simulink model "PLCCylinderCascade"  (R2020a)
settings: Solver=VariableStepAuto  StartTime=0.0  StopTime=inf  RelTol=1e-3
libraries: library_plc2simulink x27
settings Model: EnablePacing=on  Creator=Moritz  LastModifiedBy=Moritz

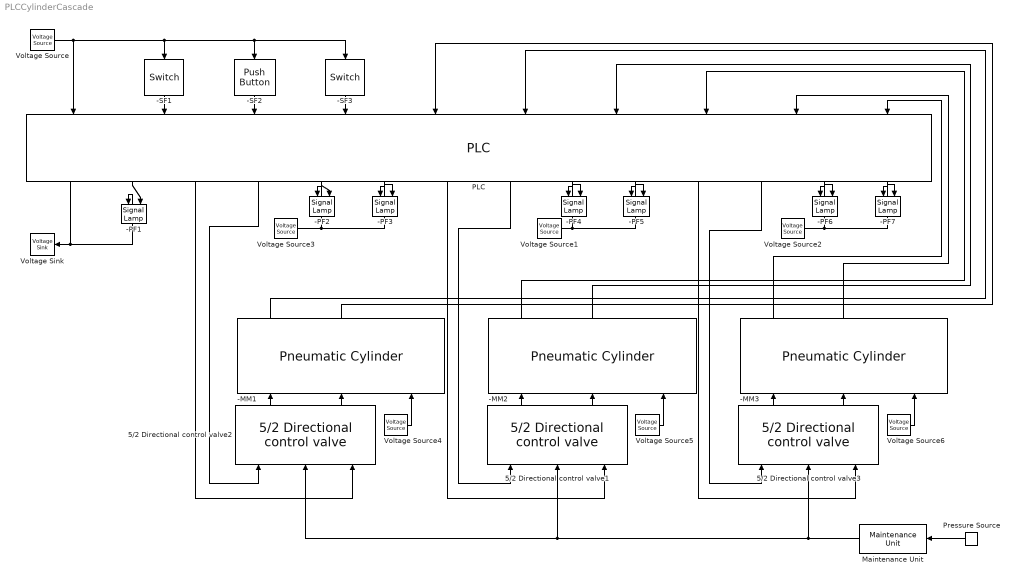
== system PLCCylinderCascade ==
  -MM1 : library_plc2simulink/Pneumatic Cylinder  minPos=0  maxPos=100  pistonSpeed=200  currentPos=-2.3002e-28  updateIcon=0.1
      settings: SourceProductName=PLC2Simulink
  -MM2 : library_plc2simulink/Pneumatic Cylinder  minPos=0  maxPos=100  pistonSpeed=200  currentPos=-2.3002e-28  updateIcon=0.1
      settings: SourceProductName=PLC2Simulink
  -MM3 : library_plc2simulink/Pneumatic Cylinder  minPos=0  maxPos=100  pistonSpeed=200  currentPos=-2.3002e-28  updateIcon=0.1
      settings: SourceProductName=PLC2Simulink
  -PF1 : library_plc2simulink/Signal Lamp  Value=off  updateTime=0.1  colorOn=[0.2,1,0.2]  colorOff=[1,1,1]
      settings: SourceProductName=PLC2Simulink
  -PF2 : library_plc2simulink/Signal Lamp  Value=on  updateTime=0.1  colorOn=[0.2,1,0.2]  colorOff=[1,1,1]
      settings: SourceProductName=PLC2Simulink
  -PF3 : library_plc2simulink/Signal Lamp  Value=off  updateTime=0.1  colorOn=[1,1,0.2]  colorOff=[1,1,1]
      settings: SourceProductName=PLC2Simulink
  -PF4 : library_plc2simulink/Signal Lamp  Value=on  updateTime=0.1  colorOn=[0.2,1,0.2]  colorOff=[1,1,1]
      settings: SourceProductName=PLC2Simulink
  -PF5 : library_plc2simulink/Signal Lamp  Value=off  updateTime=0.1  colorOn=[1,1,0.2]  colorOff=[1,1,1]
      settings: SourceProductName=PLC2Simulink
  -PF6 : library_plc2simulink/Signal Lamp  Value=on  updateTime=0.1  colorOn=[0.2,1,0.2]  colorOff=[1,1,1]
      settings: SourceProductName=PLC2Simulink
  -PF7 : library_plc2simulink/Signal Lamp  Value=off  updateTime=0.1  colorOn=[1,1,0.2]  colorOff=[1,1,1]
      settings: SourceProductName=PLC2Simulink
  -SF1 : library_plc2simulink/Switch  Gain=0  Multiplication=Element-wise(K.*u)  ParamMin=[]  ParamMax=[]  OutMin=[]  OutMax=[]  SampleTime=-1
      settings: SourceProductName=PLC2Simulink
  -SF2 : library_plc2simulink/Push Button  deactTime=0.3  StateOn=0
      settings: SourceProductName=PLC2Simulink
  -SF3 : library_plc2simulink/Switch  Gain=0  Multiplication=Element-wise(K.*u)  ParamMin=[]  ParamMax=[]  OutMin=[]  OutMax=[]  SampleTime=-1
      settings: SourceProductName=PLC2Simulink
  5/2 Directional control valve1 : library_plc2simulink/5//2 Directional control valve  updateIcon=0.1  state=0
      settings: SourceProductName=PLC2Simulink
  5/2 Directional control valve2 : library_plc2simulink/5//2 Directional control valve  updateIcon=0.1  state=0
      settings: SourceProductName=PLC2Simulink
  5/2 Directional control valve3 : library_plc2simulink/5//2 Directional control valve  updateIcon=0.1  state=0
      settings: SourceProductName=PLC2Simulink
  Maintenance Unit : library_plc2simulink/Maintenance Unit  pressure=0.300
      settings: SourceProductName=PLC2Simulink
  PLC : library_plc2simulink/PLC  instanceName=PLC1  numInputs=9  numOutputs=13  timeStep=0.05  externalSupplyVoltage=on
      settings: SourceProductName=PLC2Simulink
  Pressure Source : library_plc2simulink/Pressure Source  pressure=5
      settings: SourceProductName=PLC2Simulink
  Voltage Sink : library_plc2simulink/Voltage Sink
      settings: SourceProductName=PLC2Simulink
  Voltage Source{,4..6} (4 alike) : library_plc2simulink/Voltage Source  voltage=24
      settings: SourceProductName=PLC2Simulink
  Voltage Source1 : library_plc2simulink/Voltage Source  voltage=0
      settings: SourceProductName=PLC2Simulink
  Voltage Source2 : library_plc2simulink/Voltage Source  voltage=0
      settings: SourceProductName=PLC2Simulink
  Voltage Source3 : library_plc2simulink/Voltage Source  voltage=0
      settings: SourceProductName=PLC2Simulink
  wires:
  Pressure Source/1 -> Maintenance Unit/1
  -SF3/1 -> PLC/4
  Voltage Source/1 -> -SF3/1, -SF2/1, -SF1/1, PLC/1
  -SF1/1 -> PLC/2
  -SF2/1 -> PLC/3
  PLC/2 -> -PF1/1
  PLC/3 -> 5/2 Directional control valve2/3
  5/2 Directional control valve2/2 -> -MM1/2
  PLC/4 -> 5/2 Directional control valve2/1
  Voltage Source3/1 -> -PF3/2, -PF2/2
  5/2 Directional control valve2/1 -> -MM1/1
  PLC/6 -> -PF3/1
  PLC/5 -> -PF2/1
  5/2 Directional control valve1/2 -> -MM2/2
  5/2 Directional control valve1/1 -> -MM2/1
  PLC/8 -> 5/2 Directional control valve1/1
  PLC/7 -> 5/2 Directional control valve1/3
  Voltage Source1/1 -> -PF5/2, -PF4/2
  PLC/9 -> -PF4/1
  PLC/10 -> -PF5/1
  5/2 Directional control valve3/1 -> -MM3/1
  5/2 Directional control valve3/2 -> -MM3/2
  Voltage Source2/1 -> -PF7/2, -PF6/2
  PLC/11 -> 5/2 Directional control valve3/3
  PLC/12 -> 5/2 Directional control valve3/1
  PLC/13 -> -PF6/1
  PLC/14 -> -PF7/1
  -MM1/1 -> PLC/6
  -MM1/2 -> PLC/5
  -MM2/2 -> PLC/7
  -MM2/1 -> PLC/8
  -MM3/1 -> PLC/10
  -MM3/2 -> PLC/9
  Maintenance Unit/1 -> 5/2 Directional control valve2/2, 5/2 Directional control valve1/2, 5/2 Directional control valve3/2
  Voltage Source4/1 -> -MM1/3
  Voltage Source5/1 -> -MM2/3
  Voltage Source6/1 -> -MM3/3
  PLC/1 -> -PF1/2, Voltage Sink/1
